simulink subsystem "ScanBlockwithDC"  (R2025b)
settings: Solver=VariableStepAuto  StartTime=0.0  StopTime=10.0  RelTol=1e-3
model mask{F0=grid.frequency, Theta0=0, Kp_LF=pll.kp, Ki_LF=pll.ki, Ts=5e-5, voltage=Base.KV_base_new, voltagedc=0, mva=0, Amplitude=0, Amplitude1=0, Amplitudedc=0, f=0, T=T, Tdis=5, Tend=10, VSelect=Equivalent Series Voltage (V), Hold=Yes}
  mask prompts: F0 "physmod:ee:library:comments:control:eeSinusoidalMeasurement:InitialFrequencyHz_MP"; Theta0 "physmod:ee:library:comments:control:eeSinusoidalMeasurement:InitialPhaseAnglerad_MP"; Kp_LF "physmod:ee:library:comments:control:eeSinusoidalMeasurement:LoopFilterProportionalGain_MP"; Ki_LF "physmod:ee:library:comments:control:eeSinusoidalMeasurement:LoopFilterIntegralGain_MP"; Ts "physmod:ee:library:comments:control:eeSinusoidalMeasurement:SampleTime1ForInherited_MP"; voltage "Base Voltage AC (Volts)"; voltagedc "Base Voltage DC (Volts)"; mva "Base Volt Ampere (VA)"; Amplitude "PRBS Magnitude Along Vd (PU)"; Amplitude1 "PRBS Magnitude Along Vq (PU)"; Amplitudedc "PRBS Magnitude Along Vdc (PU)"; f "Disturbance Frequency Vector (Hz)"; T "Sample Time of PRBS (sec)"; Tdis "Injection Start Time (sec)"; Tend "Injection End Time (sec)"; VSelect "Voltage Measuremnt Point"; Hold "Hold Frequency constant During Disturbance"
undefined symbols (not defined in the file or in its folder): DiscIntNeverNeededParam, ee_sli_rtmsupport, gcbh, w
libraries: slctrl_fre x12, ee_lib x5, eeGeneralControl x4, eeTransforms x4, nesl_utility x3, slctrl_signal x3, simulink x1
(part 1 of 3)
settings Model: Creator=rajarshd  LastModifiedBy=rajarshd
settings RTWCC: GPUComputeCapability=3.5

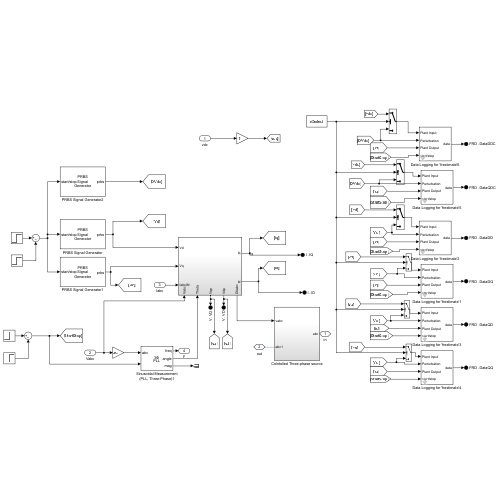
[thumbnail: Simulink's stored preview of the top-level diagram]
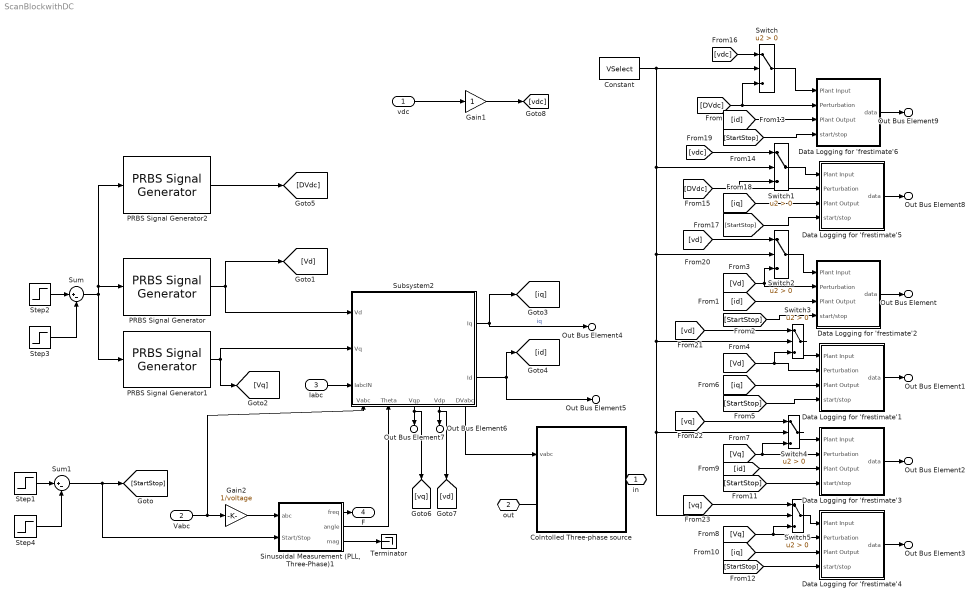
== system ScanBlockwithDC ==
  vdc : Inport
  Vabc : Inport  Port=2
  Iabc : Inport  Port=3
  Colntolled Three-phase source : Subsystem
  Constant : Constant  Value=VSelect
  Data Logging for 'frestimate'1 : Subsystem  mask(Companion Data Logger){Ts=T, SignalType=PRBS, Frequencies=[1:1:2e3], NumOfSetPeriod=1, NumOfEstPeriod=1, PRBSNumOfPeriod=1, ReadySignalActiveChoice=VariantPRBS, InfoSignalActiveChoice=VariantPRBS}
      mask prompts: Ts "Sample Time (Ts)"; SignalType "Input Signal Type"; Frequencies "Frequencies Vector"; NumOfSetPeriod "Number of Settling Periods"; NumOfEstPeriod "Number of Estimation Periods"; PRBSNumOfPeriod "Number of PRBS Signal Periods"; ReadySignalActiveChoice "Simulink:Variants:LabelComboBox"; InfoSignalActiveChoice "Simulink:Variants:LabelComboBox"
      mask help: Log data from signal generator blocks to work with "frestimate" API or frequency response estimation.
      mask init:
      | IsSinestreamSignal = strcmpi(get_param(gcb,'SignalType'),'Sinestream');
      |     IsPRBSSignal = strcmpi(get_param(gcb,'SignalType'),'PRBS');
      |     maskObj = Simulink.Mask.get(gcb);
      |     objectSinestream = maskObj.getDialogControl('SinestreamPanel');
      |     objectPRBS = maskObj.getDialogControl('PRBSPanel');
      |     %% Update optional inports
      |     inport_name = {'Frequency Index'};
      |     AvailableBlocks = get_param(gcb,'Blocks');
      |     % what exists in the block (old)
      |     type_in_block = ismember(inport_name,AvailableBlocks);
      |     % what is specified in the dialog (new)
      |     type_in_mask = IsSinestreamSignal;
      |     if IsSinestreamSignal
      |         objectSinestream.Visible = 'on';
      |         objectPRBS.Visible = 'off';
      |         set_param(gcb,'ReadySignalActiveChoice','VariantSinestream');  
      |         set_param(gcb,'InfoSignalActiveChoice','VariantSinestream');        
      |     elseif IsPRBSSignal
      |         objectSinestream.Visible = 'off';
      |         objectPRBS.Visible = 'on';
      |         set_param(gcb,'ReadySignalActiveChoice','VariantPRBS');  
      |         set_param(gcb,'InfoSignalActiveChoice','VariantPRBS');        
      |     end
      |     % Update Inport
      |     port = 5;
      |     %port = slctrlblkdlgs.OnlinePIDTuner.utilUpdateInport(gcb,'RateTransition_idx',AvailableBlocks,type_in_mask,type_in_block,1,'Frequency Index',port,1,'Frequencies','double');
      mask TypeOptions SignalType: Sinestream | PRBS
      mask TypeOptions ReadySignalActiveChoice: Generate Ready Signal/LabelModeActiveChoice
      mask TypeOptions InfoSignalActiveChoice: Generate Info Signal/LabelModeActiveChoice
      mask DialogControl Container3 Prompt: Signal Specific Settings
      mask DialogControl ReadySignalActiveChoice Prompt: Label mode active choice:
      mask DialogControl InfoSignalActiveChoice Prompt: Label mode active choice:
  Data Logging for 'frestimate'2 : Subsystem  mask(Companion Data Logger){Ts=T, SignalType=PRBS, Frequencies=[1:1:2e3], NumOfSetPeriod=1, NumOfEstPeriod=1, PRBSNumOfPeriod=1, ReadySignalActiveChoice=VariantPRBS, InfoSignalActiveChoice=VariantPRBS}
      mask prompts: Ts "Sample Time (Ts)"; SignalType "Input Signal Type"; Frequencies "Frequencies Vector"; NumOfSetPeriod "Number of Settling Periods"; NumOfEstPeriod "Number of Estimation Periods"; PRBSNumOfPeriod "Number of PRBS Signal Periods"; ReadySignalActiveChoice "Simulink:Variants:LabelComboBox"; InfoSignalActiveChoice "Simulink:Variants:LabelComboBox"
      mask help: Log data from signal generator blocks to work with "frestimate" API or frequency response estimation.
      mask init:
      | IsSinestreamSignal = strcmpi(get_param(gcb,'SignalType'),'Sinestream');
      |     IsPRBSSignal = strcmpi(get_param(gcb,'SignalType'),'PRBS');
      |     maskObj = Simulink.Mask.get(gcb);
      |     objectSinestream = maskObj.getDialogControl('SinestreamPanel');
      |     objectPRBS = maskObj.getDialogControl('PRBSPanel');
      |     %% Update optional inports
      |     inport_name = {'Frequency Index'};
      |     AvailableBlocks = get_param(gcb,'Blocks');
      |     % what exists in the block (old)
      |     type_in_block = ismember(inport_name,AvailableBlocks);
      |     % what is specified in the dialog (new)
      |     type_in_mask = IsSinestreamSignal;
      |     if IsSinestreamSignal
      |         objectSinestream.Visible = 'on';
      |         objectPRBS.Visible = 'off';
      |         set_param(gcb,'ReadySignalActiveChoice','VariantSinestream');  
      |         set_param(gcb,'InfoSignalActiveChoice','VariantSinestream');        
      |     elseif IsPRBSSignal
      |         objectSinestream.Visible = 'off';
      |         objectPRBS.Visible = 'on';
      |         set_param(gcb,'ReadySignalActiveChoice','VariantPRBS');  
      |         set_param(gcb,'InfoSignalActiveChoice','VariantPRBS');        
      |     end
      |     % Update Inport
      |     port = 5;
      |   %  port = slctrlblkdlgs.OnlinePIDTuner.utilUpdateInport(gcb,'RateTransition_idx',AvailableBlocks,type_in_mask,type_in_block,1,'Frequency Index',port,1,'Frequencies','double');
      mask TypeOptions SignalType: Sinestream | PRBS
      mask TypeOptions ReadySignalActiveChoice: Generate Ready Signal/LabelModeActiveChoice
      mask TypeOptions InfoSignalActiveChoice: Generate Info Signal/LabelModeActiveChoice
      mask DialogControl Container3 Prompt: Signal Specific Settings
      mask DialogControl ReadySignalActiveChoice Prompt: Label mode active choice:
      mask DialogControl InfoSignalActiveChoice Prompt: Label mode active choice:
  Data Logging for 'frestimate'3 : Subsystem  mask(Companion Data Logger){Ts=T, SignalType=PRBS, Frequencies=[1:1:2e3], NumOfSetPeriod=1, NumOfEstPeriod=1, PRBSNumOfPeriod=1, ReadySignalActiveChoice=VariantPRBS, InfoSignalActiveChoice=VariantPRBS}
      mask prompts: Ts "Sample Time (Ts)"; SignalType "Input Signal Type"; Frequencies "Frequencies Vector"; NumOfSetPeriod "Number of Settling Periods"; NumOfEstPeriod "Number of Estimation Periods"; PRBSNumOfPeriod "Number of PRBS Signal Periods"; ReadySignalActiveChoice "Simulink:Variants:LabelComboBox"; InfoSignalActiveChoice "Simulink:Variants:LabelComboBox"
      mask help: Log data from signal generator blocks to work with "frestimate" API or frequency response estimation.
      mask init: same as ScanBlockwithDC/Data Logging for 'frestimate'1
      mask TypeOptions SignalType: Sinestream | PRBS
      mask TypeOptions ReadySignalActiveChoice: Generate Ready Signal/LabelModeActiveChoice
      mask TypeOptions InfoSignalActiveChoice: Generate Info Signal/LabelModeActiveChoice
      mask DialogControl Container3 Prompt: Signal Specific Settings
      mask DialogControl ReadySignalActiveChoice Prompt: Label mode active choice:
      mask DialogControl InfoSignalActiveChoice Prompt: Label mode active choice:
  Data Logging for 'frestimate'4 : Subsystem  mask(Companion Data Logger){Ts=T, SignalType=PRBS, Frequencies=[1:1:2e3], NumOfSetPeriod=1, NumOfEstPeriod=1, PRBSNumOfPeriod=1, ReadySignalActiveChoice=VariantPRBS, InfoSignalActiveChoice=VariantPRBS}
      mask prompts: Ts "Sample Time (Ts)"; SignalType "Input Signal Type"; Frequencies "Frequencies Vector"; NumOfSetPeriod "Number of Settling Periods"; NumOfEstPeriod "Number of Estimation Periods"; PRBSNumOfPeriod "Number of PRBS Signal Periods"; ReadySignalActiveChoice "Simulink:Variants:LabelComboBox"; InfoSignalActiveChoice "Simulink:Variants:LabelComboBox"
      mask help: Log data from signal generator blocks to work with "frestimate" API or frequency response estimation.
      mask init: same as ScanBlockwithDC/Data Logging for 'frestimate'1
      mask TypeOptions SignalType: Sinestream | PRBS
      mask TypeOptions ReadySignalActiveChoice: Generate Ready Signal/LabelModeActiveChoice
      mask TypeOptions InfoSignalActiveChoice: Generate Info Signal/LabelModeActiveChoice
      mask DialogControl Container3 Prompt: Signal Specific Settings
      mask DialogControl ReadySignalActiveChoice Prompt: Label mode active choice:
      mask DialogControl InfoSignalActiveChoice Prompt: Label mode active choice:
  Data Logging for 'frestimate'5 : Subsystem  mask(Companion Data Logger){Ts=T, SignalType=PRBS, Frequencies=[1:1:2e3], NumOfSetPeriod=1, NumOfEstPeriod=1, PRBSNumOfPeriod=1, ReadySignalActiveChoice=VariantPRBS, InfoSignalActiveChoice=VariantPRBS}
      mask prompts: Ts "Sample Time (Ts)"; SignalType "Input Signal Type"; Frequencies "Frequencies Vector"; NumOfSetPeriod "Number of Settling Periods"; NumOfEstPeriod "Number of Estimation Periods"; PRBSNumOfPeriod "Number of PRBS Signal Periods"; ReadySignalActiveChoice "Simulink:Variants:LabelComboBox"; InfoSignalActiveChoice "Simulink:Variants:LabelComboBox"
      mask help: Log data from signal generator blocks to work with "frestimate" API or frequency response estimation.
      mask init:
      | IsSinestreamSignal = strcmpi(get_param(gcb,'SignalType'),'Sinestream');
      |     IsPRBSSignal = strcmpi(get_param(gcb,'SignalType'),'PRBS');
      |     maskObj = Simulink.Mask.get(gcb);
      |     objectSinestream = maskObj.getDialogControl('SinestreamPanel');
      |     objectPRBS = maskObj.getDialogControl('PRBSPanel');
      |     %% Update optional inports
      |     inport_name = {'Frequency Index'};
      |     AvailableBlocks = get_param(gcb,'Blocks');
      |     % what exists in the block (old)
      |     type_in_block = ismember(inport_name,AvailableBlocks);
      |     % what is specified in the dialog (new)
      |     type_in_mask = IsSinestreamSignal;
      |     if IsSinestreamSignal
      |         objectSinestream.Visible = 'on';
      |         objectPRBS.Visible = 'off';
      |         set_param(gcb,'ReadySignalActiveChoice','VariantSinestream');  
      |         set_param(gcb,'InfoSignalActiveChoice','VariantSinestream');        
      |     elseif IsPRBSSignal
      |         objectSinestream.Visible = 'off';
      |         objectPRBS.Visible = 'on';
      |         set_param(gcb,'ReadySignalActiveChoice','VariantPRBS');  
      |         set_param(gcb,'InfoSignalActiveChoice','VariantPRBS');        
      |     end
      |     % Update Inport
      |     port = 5;
      |    % port = slctrlblkdlgs.OnlinePIDTuner.utilUpdateInport(gcb,'RateTransition_idx',AvailableBlocks,type_in_mask,type_in_block,1,'Frequency Index',port,1,'Frequencies','double');
      mask TypeOptions SignalType: Sinestream | PRBS
      mask TypeOptions ReadySignalActiveChoice: Generate Ready Signal/LabelModeActiveChoice
      mask TypeOptions InfoSignalActiveChoice: Generate Info Signal/LabelModeActiveChoice
      mask DialogControl Container3 Prompt: Signal Specific Settings
      mask DialogControl ReadySignalActiveChoice Prompt: Label mode active choice:
      mask DialogControl InfoSignalActiveChoice Prompt: Label mode active choice:
  Data Logging for 'frestimate'6 : Subsystem  mask(Companion Data Logger){Ts=T, SignalType=PRBS, Frequencies=[1:1:2e3], NumOfSetPeriod=1, NumOfEstPeriod=1, PRBSNumOfPeriod=1, ReadySignalActiveChoice=VariantPRBS, InfoSignalActiveChoice=VariantPRBS}
      mask prompts: Ts "Sample Time (Ts)"; SignalType "Input Signal Type"; Frequencies "Frequencies Vector"; NumOfSetPeriod "Number of Settling Periods"; NumOfEstPeriod "Number of Estimation Periods"; PRBSNumOfPeriod "Number of PRBS Signal Periods"; ReadySignalActiveChoice "Simulink:Variants:LabelComboBox"; InfoSignalActiveChoice "Simulink:Variants:LabelComboBox"
      mask help: Log data from signal generator blocks to work with "frestimate" API or frequency response estimation.
      mask init: same as ScanBlockwithDC/Data Logging for 'frestimate'5
      mask TypeOptions SignalType: Sinestream | PRBS
      mask TypeOptions ReadySignalActiveChoice: Generate Ready Signal/LabelModeActiveChoice
      mask TypeOptions InfoSignalActiveChoice: Generate Info Signal/LabelModeActiveChoice
      mask DialogControl Container3 Prompt: Signal Specific Settings
      mask DialogControl ReadySignalActiveChoice Prompt: Label mode active choice:
      mask DialogControl InfoSignalActiveChoice Prompt: Label mode active choice:
  Gain1 : Gain
  Gain2 : Gain  Gain=1/voltage
  PRBS Signal Generator : slctrl_signal/PRBS Signal Generator  DiscreteTs=T  BlockDataType=double  SignalSource=Block parameters  Frequencies=f*2*pi  FreqUnits=rad/s  Amplitudes=Amplitude*voltage+1e-9  NumOfFreq=3  NumOfPRBSPeriod=1  UseAutogenNumOfPRBSPeriod=off  PRBSSignalOrder=16  UseAutogenPRBSSignalOrder=on  UseExternalTs=off  CompiledTsChoice=InternalTs
      settings: LibrarySourceBlock=slctrlblks/Signal Generation/PRBS Signal Generator
  PRBS Signal Generator1 : slctrl_signal/PRBS Signal Generator  DiscreteTs=T  BlockDataType=double  SignalSource=Block parameters  Frequencies=f*2*pi  FreqUnits=rad/s  Amplitudes=Amplitude1*voltage+1e-9  NumOfFreq=3  NumOfPRBSPeriod=1  UseAutogenNumOfPRBSPeriod=off  PRBSSignalOrder=16  UseAutogenPRBSSignalOrder=on  UseExternalTs=off  CompiledTsChoice=InternalTs
      settings: LibrarySourceBlock=slctrlblks/Signal Generation/PRBS Signal Generator
  PRBS Signal Generator2 : slctrl_signal/PRBS Signal Generator  DiscreteTs=T  BlockDataType=double  SignalSource=Block parameters  Frequencies=f*2*pi  FreqUnits=rad/s  Amplitudes=Amplitudedc*voltagedc+1e-9  NumOfFreq=3  NumOfPRBSPeriod=1  UseAutogenNumOfPRBSPeriod=off  PRBSSignalOrder=16  UseAutogenPRBSSignalOrder=on  UseExternalTs=off  CompiledTsChoice=InternalTs
      settings: LibrarySourceBlock=slctrlblks/Signal Generation/PRBS Signal Generator
  "Sinusoidal Measurement (PLL, Three-Phase)1" : Subsystem  LoadFcn=ee_sli_rtmsupport( 'loadfcn', gcbh );  mask(Sinusoidal Measurement (PLL, Three-Phase)){Kp_LF=Kp_LF, Ki_LF=Ki_LF, F0=F0, Theta0=Theta0, Ts=Ts}
      mask prompts: Kp_LF "physmod:ee:library:comments:control:eeSinusoidalMeasurement:LoopFilterProportionalGain_MP"; Ki_LF "physmod:ee:library:comments:control:eeSinusoidalMeasurement:LoopFilterIntegralGain_MP"; F0 "physmod:ee:library:comments:control:eeSinusoidalMeasurement:InitialFrequencyHz_MP"; Theta0 "physmod:ee:library:comments:control:eeSinusoidalMeasurement:InitialPhaseAnglerad_MP"; Ts "physmod:ee:library:comments:control:eeSinusoidalMeasurement:SampleTime1ForInherited_MP"
      mask help: physmod:ee:library:comments:control:eeSinusoidalMeasurement:SinusoidalPowerMeasurementPLLThreePhase_MD
      mask init:
      | timeDomain = ee.mask.initializeThreePhaseSinusoidalMeasurementPLL(Ts);
      settings: CopyFcn=ee_sli_rtmsupport( 'copyfcn', gcbh );  DeleteFcn=ee_sli_rtmsupport( 'deletefcn', gcbh );  ModelCloseFcn=ee_sli_rtmsupport( 'modelclosefcn', gcbh );  PostSaveFcn=ee_sli_rtmsupport( 'postsavefcn', gcbh );  PreCopyFcn=ee_sli_rtmsupport( 'precopyfcn', gcbh );  OpenFcn=ee_sli_rtmsupport( 'openfcn', gcbh );  CloseFcn=ee_sli_rtmsupport( 'closefcn', gcbh );  PreDeleteFcn=ee_sli_rtmsupport( 'predeletefcn', gcbh );
      settings: LibrarySourceBlock=|
      | ee_sl_lib/Measurements/Sinusoidal Measurement
      | (PLL, Three-Phase)
      mask Help: web(nesl_help(gcbh))
      mask TypeOptions Ts:
      | Angle/Integrator with
      | Wrapped State
      | (Discrete or Continuous)/Ts | PI/Integrator
      | (Discrete or Continuous)/Ts | Moving Average
      | (Variable Frequency)/Ts | Low-Pass Filter
      | (Discrete or Continuous)/Ts
      mask DialogControl Kp_LF Prompt: Loop filter proportional gain
      mask DialogControl Ki_LF Prompt: Loop filter integral gain
      mask DialogControl F0 Prompt: Initial frequency (Hz)
      mask DialogControl Theta0 Prompt: Initial phase angle (rad)
      mask DialogControl Ts Prompt: Sample time (-1 for inherited)
      mask Display: ee.mask.drawThreePhaseSinusoidalMeasurementPLL;
  Step1 : Step  Time=Tdis-0.001  SampleTime=Ts
  Step2 : Step  Time=Tdis  SampleTime=Ts
  Step3 : Step  Time=Tend  SampleTime=Ts
  Step4 : Step  Time=Tend-0.001  SampleTime=Ts
  Subsystem2 : Subsystem
      settings: PortSchema="{\"entries\":[{\"content\":{\"sides\":[{\"content\":{\"connectorIds\":[\"In1\",\"In2\",\"In3\"]},\"type\":\"ConnectorPlacement.EquallySpacedRectSide\",\"uuid\":\"9594ab20-6a90-4061-9191-964719779161\"},{\"content\":{\"connectorIds\":[\"Out1\",\"Out2\"],\"side\":\"RIGHT\"},\"type\":\"ConnectorPlacement.EquallySpacedRectSide\",\"uuid\":\"7728c146-30c2-48f5-81ca-653b56ee64fb\"},{\"content\":{\"side\":\"TOP\"},\"type\":\"ConnectorPlacement.EquallySpacedRectSide\",\"uuid\":\"8060c2dd-01d9-4157-a0b3-59db77887fcf\"},{\"content\":{\"connectorIds\":[\"In4\",\"In5\",\"Out3\",\"Out4\",\"Out5\"],\"side\":\"BOTTOM\"},\"type\":\"ConnectorPlacement.EquallySpacedRectSide\",\"uuid\":\"6c62adf9-210a-4ad7-b383-6cff41840c61\"}]},\"type\":\"ConnectorPlacement.EquallySpacedConnector\",\"uuid\":\"38a4dacf-dba1-4794-be83-b6cd11059d5d\"}],\"packageUris\":[\"http://schema.mathworks.com/mf0/Connector/R2020b\"],\"version\":\"1.0\"}"
  Sum : Sum  Inputs=|+-
  Sum1 : Sum  Inputs=|+-
  Switch{,1..5} (6 alike) : Switch  Criteria=u2 > Threshold  SaturateOnIntegerOverflow=off  InputSameDT=off
  Terminator : Terminator
  in : PMIOPort  Side=Left
  out : PMIOPort  Port=2  Side=Right
  Out Bus Element : Outport  PortName=FRD  Element=DataDD
  Out Bus Element1 : Outport  PortName=FRD  Element=DataDQ
  Out Bus Element2 : Outport  PortName=FRD  Element=DataQD
  Out Bus Element3 : Outport  PortName=FRD  Element=DataQQ
  Out Bus Element8 : Outport  PortName=FRD  Element=DataQDC
  Out Bus Element9 : Outport  PortName=FRD  Element=DataDDC
  Out Bus Element4 : Outport  Port=2  PortName=I  Element=IQ
  Out Bus Element5 : Outport  Port=2  PortName=I  Element=ID
  Out Bus Element6 : Outport  Port=3  PortName=V  Element=VD
  Out Bus Element7 : Outport  Port=3  PortName=V  Element=VQ
  F : Outport  Port=4  SampleTime=Ts
  wires:
  PRBS Signal Generator1/1 -> Subsystem2/2(Vq), [Vq]
  "Sinusoidal Measurement (PLL, Three-Phase)1"/1(freq) -> F/1
  Subsystem2/5(DVabc) -> Colntolled Three-phase source/1(vabc)
  "Sinusoidal Measurement (PLL, Three-Phase)1"/2(angle) -> Subsystem2/5(Theta)
  Subsystem2/1(Iq) -> [iq], Out Bus Element4/1  "iq"
  Subsystem2/2(Id) -> [id], Out Bus Element5/1
  "Sinusoidal Measurement (PLL, Three-Phase)1"/3(mag) -> Terminator/1
  Step2/1 -> Sum/1
  Sum/1 -> PRBS Signal Generator1/1, PRBS Signal Generator/1, PRBS Signal Generator2/1
  Step3/1 -> Sum/2
  PRBS Signal Generator/1 -> Subsystem2/1(Vd), [Vd]
  [id] -> Data Logging for 'frestimate'2/3(Plant Output)
  [StartStop] -> Data Logging for 'frestimate'2/4(start/stop)
  [StartStop] -> Data Logging for 'frestimate'1/4(start/stop)
  [iq] -> Data Logging for 'frestimate'1/3(Plant Output)
  [id] -> Data Logging for 'frestimate'3/3(Plant Output)
  [iq] -> Data Logging for 'frestimate'4/3(Plant Output)
  [StartStop] -> Data Logging for 'frestimate'3/4(start/stop)
  [StartStop] -> Data Logging for 'frestimate'4/4(start/stop)
  Step4/1 -> Sum1/2
  Step1/1 -> Sum1/1
  Subsystem2/4(Vdp) -> Out Bus Element6/1, [vd]
  Subsystem2/3(Vqp) -> Out Bus Element7/1, [vq]
  Iabc/1 -> Subsystem2/3(IabcIN)
  Data Logging for 'frestimate'2/1(data) -> Out Bus Element/1
  Data Logging for 'frestimate'1/1(data) -> Out Bus Element1/1
  Data Logging for 'frestimate'3/1(data) -> Out Bus Element2/1
  Data Logging for 'frestimate'4/1(data) -> Out Bus Element3/1
  Sum1/1 -> [StartStop], "Sinusoidal Measurement (PLL, Three-Phase)1"/2(Start/Stop)
  Data Logging for 'frestimate'5/1(data) -> Out Bus Element8/1
  Data Logging for 'frestimate'6/1(data) -> Out Bus Element9/1
  [iq] -> Data Logging for 'frestimate'5/3(Plant Output)
  [StartStop] -> Data Logging for 'frestimate'5/4(start/stop)
  [id] -> Data Logging for 'frestimate'6/3(Plant Output)
  [StartStop] -> Data Logging for 'frestimate'6/4(start/stop)
  PRBS Signal Generator2/1 -> [DVdc]
  [DVdc] -> Data Logging for 'frestimate'6/2(Perturbation), Switch/3
  [DVdc] -> Data Logging for 'frestimate'5/2(Perturbation), Switch1/3
  vdc/1 -> Gain1/1
  [Vd] -> Switch2/3, Data Logging for 'frestimate'2/2(Perturbation)
  [Vd] -> Data Logging for 'frestimate'1/2(Perturbation), Switch3/3
  [Vq] -> Data Logging for 'frestimate'3/2(Perturbation), Switch4/3
  [Vq] -> Data Logging for 'frestimate'4/2(Perturbation), Switch5/3
  Vabc/1 -> Subsystem2/4(Vabc), Gain2/1
  Gain1/1 -> [vdc]
  Gain2/1 -> "Sinusoidal Measurement (PLL, Three-Phase)1"/1(abc)
  [vdc] -> Switch/1
  Switch/1 -> Data Logging for 'frestimate'6/1(Plant Input)
  Switch1/1 -> Data Logging for 'frestimate'5/1(Plant Input)
  [vdc] -> Switch1/1
  Constant/1 -> Switch/2, Switch1/2, Switch3/2, Switch5/2, Switch4/2, Switch2/2
  [vd] -> Switch2/1
  Switch2/1 -> Data Logging for 'frestimate'2/1(Plant Input)
  Switch3/1 -> Data Logging for 'frestimate'1/1(Plant Input)
  [vd] -> Switch3/1
  Switch4/1 -> Data Logging for 'frestimate'3/1(Plant Input)
  [vq] -> Switch4/1
  Switch5/1 -> Data Logging for 'frestimate'4/1(Plant Input)
  [vq] -> Switch5/1
  connections:
  Colntolled Three-phase source/RConn1 -- in/RConn1
  out/RConn1 -- Colntolled Three-phase source/LConn1

== system ScanBlockwithDC/Colntolled Three-phase source ==
  vabc : Inport
  Demux : Demux  Outputs=3
  Phase Splitter : ee_lib/Connectors & References/Phase Splitter
  Phase Splitter1 : ee_lib/Connectors & References/Phase Splitter
  Programmable Voltage Source : ee_lib/Sources/Programmable Voltage Source  magnitude_type=ee.enum.timechanging.constant  ac_magnitude=0 V  magn_ramp=1 V/s  magn_step=1 V  magn_modu_magn=1 V  magn_modu_freq=1 Hz  magn_t1=1 s  magn_t2=2 s  frequency_type=ee.enum.timechanging.constant  ac_frequency=60 Hz  freq_ramp=1 Hz/s  freq_step=1 Hz  freq_modu_magn=1 Hz  freq_modu_freq=1 Hz  freq_t1=1 s  freq_t2=2 s  phase_type=ee.enum.timechanging.constant  ac_shift=0 deg  phase_ramp=1 deg/s  phase_step=1 deg  phase_modu_magn=1 deg  phase_modu_freq=1 Hz  phase_t1=1 s  phase_t2=2 s  dc_type=ee.enum.timechanging.external  dc_voltage=0 V  dc_ramp=1 V/s  dc_step=1 V  dc_modu_magn=1 V  dc_modu_freq=1 Hz  dc_t1=1 s  dc_t2=2 s  harmonic_option=0  harmonic_orders=[5, 7, 11, 13]  harmonic_ratios=[.1, .1, .1, .1]  harmonic_shifts=[0, 0, 0, 0] deg  harmonic_t1=-inf s  harmonic_t2=inf s  noise_mode=0  PSD=0 V^2/Hz  repeatability=1  auto_seed=0  user_seed=0  sample_time=1e-3 s  i_specify=off  i_priority=None  i=0 A  i_nominal_specify=off  i_nominal_value=1  i_nominal_unit=A  v_specify=off  v_priority=None  v=0 V  v_nominal_specify=off  v_nominal_value=1  v_nominal_unit=V
      settings: InternalSimscapePortConfiguration="{\"Bottom\":[],\"Left\":[{\"id\":\"p\",\"label\":\"+\",\"type\":\"foundation.electrical.electrical\"}],\"Right\":[{\"id\":\"ext_dc\",\"label\":\"DC\",\"type\":\"input\"},{\"id\":\"n\",\"label\":\"-\",\"type\":\"foundation.electrical.electrical\"}],\"Top\":[]}"
  Programmable Voltage Source1 : ee_lib/Sources/Programmable Voltage Source  magnitude_type=ee.enum.timechanging.constant  ac_magnitude=0 V  magn_ramp=1 V/s  magn_step=1 V  magn_modu_magn=1 V  magn_modu_freq=1 Hz  magn_t1=1 s  magn_t2=2 s  frequency_type=ee.enum.timechanging.constant  ac_frequency=60 Hz  freq_ramp=1 Hz/s  freq_step=1 Hz  freq_modu_magn=1 Hz  freq_modu_freq=1 Hz  freq_t1=1 s  freq_t2=2 s  phase_type=ee.enum.timechanging.constant  ac_shift=0 deg  phase_ramp=1 deg/s  phase_step=1 deg  phase_modu_magn=1 deg  phase_modu_freq=1 Hz  phase_t1=1 s  phase_t2=2 s  dc_type=ee.enum.timechanging.external  dc_voltage=0 V  dc_ramp=1 V/s  dc_step=1 V  dc_modu_magn=1 V  dc_modu_freq=1 Hz  dc_t1=1 s  dc_t2=2 s  harmonic_option=0  harmonic_orders=[5, 7, 11, 13]  harmonic_ratios=[.1, .1, .1, .1]  harmonic_shifts=[0, 0, 0, 0] deg  harmonic_t1=-inf s  harmonic_t2=inf s  noise_mode=0  PSD=0 V^2/Hz  repeatability=1  auto_seed=0  user_seed=0  sample_time=1e-3 s  i_specify=off  i_priority=None  i=0 A  i_nominal_specify=off  i_nominal_value=1  i_nominal_unit=A  v_specify=off  v_priority=None  v=0 V  v_nominal_specify=off  v_nominal_value=1  v_nominal_unit=V
      settings: InternalSimscapePortConfiguration="{\"Bottom\":[],\"Left\":[{\"id\":\"p\",\"label\":\"+\",\"type\":\"foundation.electrical.electrical\"}],\"Right\":[{\"id\":\"ext_dc\",\"label\":\"DC\",\"type\":\"input\"},{\"id\":\"n\",\"label\":\"-\",\"type\":\"foundation.electrical.electrical\"}],\"Top\":[]}"
  Programmable Voltage Source2 : ee_lib/Sources/Programmable Voltage Source  magnitude_type=ee.enum.timechanging.constant  ac_magnitude=0 V  magn_ramp=1 V/s  magn_step=1 V  magn_modu_magn=1 V  magn_modu_freq=1 Hz  magn_t1=1 s  magn_t2=2 s  frequency_type=ee.enum.timechanging.constant  ac_frequency=60 Hz  freq_ramp=1 Hz/s  freq_step=1 Hz  freq_modu_magn=1 Hz  freq_modu_freq=1 Hz  freq_t1=1 s  freq_t2=2 s  phase_type=ee.enum.timechanging.constant  ac_shift=0 deg  phase_ramp=1 deg/s  phase_step=1 deg  phase_modu_magn=1 deg  phase_modu_freq=1 Hz  phase_t1=1 s  phase_t2=2 s  dc_type=ee.enum.timechanging.external  dc_voltage=0 V  dc_ramp=1 V/s  dc_step=1 V  dc_modu_magn=1 V  dc_modu_freq=1 Hz  dc_t1=1 s  dc_t2=2 s  harmonic_option=0  harmonic_orders=[5, 7, 11, 13]  harmonic_ratios=[.1, .1, .1, .1]  harmonic_shifts=[0, 0, 0, 0] deg  harmonic_t1=-inf s  harmonic_t2=inf s  noise_mode=0  PSD=0 V^2/Hz  repeatability=1  auto_seed=0  user_seed=0  sample_time=1e-3 s  i_specify=off  i_priority=None  i=0 A  i_nominal_specify=off  i_nominal_value=1  i_nominal_unit=A  v_specify=off  v_priority=None  v=0 V  v_nominal_specify=off  v_nominal_value=1  v_nominal_unit=V
      settings: InternalSimscapePortConfiguration="{\"Bottom\":[],\"Left\":[{\"id\":\"p\",\"label\":\"+\",\"type\":\"foundation.electrical.electrical\"}],\"Right\":[{\"id\":\"ext_dc\",\"label\":\"DC\",\"type\":\"input\"},{\"id\":\"n\",\"label\":\"-\",\"type\":\"foundation.electrical.electrical\"}],\"Top\":[]}"
  Simulink-PS Converter : nesl_utility/Simulink-PS Converter  PhysicalDomain=network_engine_domain  SubClassName=ps_input  LeftPortType=input  RightPortType=output  PseudoPeriodic=off  Frequencies=[]  NoiseDistribution=none  NoiseParameters=[]  Unit=1  AffineConversion=off  FilteringAndDerivatives=provide  SimscapeFilterOrder=1  InputFilterTimeConstant=0.001  UdotUserProvided=0
  Simulink-PS Converter1 : nesl_utility/Simulink-PS Converter  PhysicalDomain=network_engine_domain  SubClassName=ps_input  LeftPortType=input  RightPortType=output  PseudoPeriodic=off  Frequencies=[]  NoiseDistribution=none  NoiseParameters=[]  Unit=1  AffineConversion=off  FilteringAndDerivatives=provide  SimscapeFilterOrder=1  InputFilterTimeConstant=0.001  UdotUserProvided=0
  Simulink-PS Converter2 : nesl_utility/Simulink-PS Converter  PhysicalDomain=network_engine_domain  SubClassName=ps_input  LeftPortType=input  RightPortType=output  PseudoPeriodic=off  Frequencies=[]  NoiseDistribution=none  NoiseParameters=[]  Unit=1  AffineConversion=off  FilteringAndDerivatives=provide  SimscapeFilterOrder=1  InputFilterTimeConstant=0.001  UdotUserProvided=0
  abc1 : PMIOPort  Side=Left
  abc : PMIOPort  Port=2  Side=Right
  wires:
  Demux/1 -> Simulink-PS Converter2/1
  Demux/2 -> Simulink-PS Converter1/1
  Demux/3 -> Simulink-PS Converter/1
  vabc/1 -> Demux/1
  connections:
  abc1/RConn1 -- Phase Splitter/LConn1
  Simulink-PS Converter2/RConn1 -- Programmable Voltage Source/RConn1
  Simulink-PS Converter1/RConn1 -- Programmable Voltage Source1/RConn1
  Simulink-PS Converter/RConn1 -- Programmable Voltage Source2/RConn1
  Phase Splitter1/LConn1 -- abc/RConn1
  Programmable Voltage Source1/RConn2 -- Phase Splitter1/RConn2
  Programmable Voltage Source1/LConn1 -- Phase Splitter/RConn2
  Programmable Voltage Source/LConn1 -- Phase Splitter/RConn1
  Programmable Voltage Source/RConn2 -- Phase Splitter1/RConn1
  Programmable Voltage Source2/RConn2 -- Phase Splitter1/RConn3
  Programmable Voltage Source2/LConn1 -- Phase Splitter/RConn3

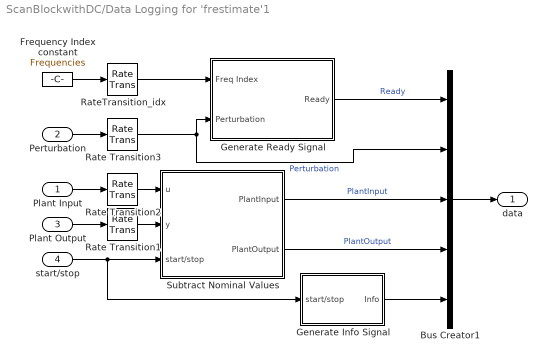
== system ScanBlockwithDC/Data Logging for 'frestimate'1 ==
  Plant Input : Inport
  Perturbation : Inport  Port=2
  Plant Output : Inport  Port=3
  start/stop : Inport  Port=4
  Bus Creator1 : BusCreator  Inputs=5
  Frequency Index constant : Constant  Value=Frequencies  OutDataTypeStr=double
  Generate Info Signal : Subsystem  Variant=on  VariantControlMode=label  LabelModeActiveChoice=VariantPRBS
  Generate Ready Signal : Subsystem  Variant=on  VariantControlMode=label  LabelModeActiveChoice=VariantPRBS
  Rate Transition1 : RateTransition  OutPortSampleTime=Ts
  Rate Transition2 : RateTransition  OutPortSampleTime=Ts
  Rate Transition3 : RateTransition  OutPortSampleTime=Ts
  RateTransition_idx : RateTransition  OutPortSampleTime=Ts
  Subtract Nominal Values : Subsystem
  data : Outport
  wires:
  Frequency Index constant/1 -> RateTransition_idx/1
  RateTransition_idx/1 -> Generate Ready Signal/1(Freq Index)
  Perturbation/1 -> Rate Transition3/1
  Rate Transition1/1 -> Subtract Nominal Values/2(y)
  Rate Transition2/1 -> Subtract Nominal Values/1(u)
  start/stop/1 -> Subtract Nominal Values/3(start/stop), Generate Info Signal/1(start/stop)
  Plant Input/1 -> Rate Transition2/1
  Plant Output/1 -> Rate Transition1/1
  Generate Ready Signal/1(Ready) -> Bus Creator1/1  "Ready"
  Subtract Nominal Values/2(PlantOutput) -> Bus Creator1/4  "PlantOutput"
  Subtract Nominal Values/1(PlantInput) -> Bus Creator1/3  "PlantInput"
  Rate Transition3/1 -> Bus Creator1/2, Generate Ready Signal/2(Perturbation)  "Perturbation"
  Bus Creator1/1 -> data/1
  Generate Info Signal/1(Info) -> Bus Creator1/5

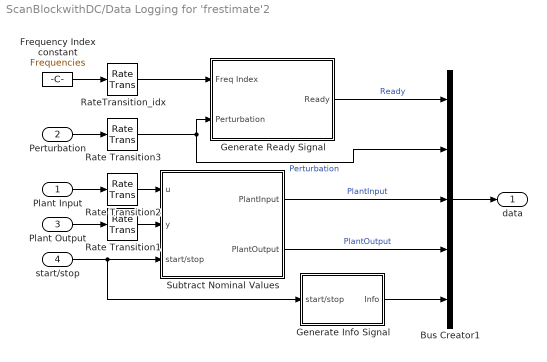
== system ScanBlockwithDC/Data Logging for 'frestimate'2 ==
  Plant Input : Inport
  Perturbation : Inport  Port=2
  Plant Output : Inport  Port=3
  start/stop : Inport  Port=4
  Bus Creator1 : BusCreator  Inputs=5
  Frequency Index constant : Constant  Value=Frequencies  OutDataTypeStr=double
  Generate Info Signal : Subsystem  Variant=on  VariantControlMode=label  LabelModeActiveChoice=VariantPRBS
  Generate Ready Signal : Subsystem  Variant=on  VariantControlMode=label  LabelModeActiveChoice=VariantPRBS
  Rate Transition1 : RateTransition  OutPortSampleTime=Ts
  Rate Transition2 : RateTransition  OutPortSampleTime=Ts
  Rate Transition3 : RateTransition  OutPortSampleTime=Ts
  RateTransition_idx : RateTransition  OutPortSampleTime=Ts
  Subtract Nominal Values : Subsystem
  data : Outport
  wires:
  Frequency Index constant/1 -> RateTransition_idx/1
  RateTransition_idx/1 -> Generate Ready Signal/1(Freq Index)
  Perturbation/1 -> Rate Transition3/1
  Rate Transition1/1 -> Subtract Nominal Values/2(y)
  Rate Transition2/1 -> Subtract Nominal Values/1(u)
  start/stop/1 -> Subtract Nominal Values/3(start/stop), Generate Info Signal/1(start/stop)
  Plant Input/1 -> Rate Transition2/1
  Plant Output/1 -> Rate Transition1/1
  Generate Ready Signal/1(Ready) -> Bus Creator1/1  "Ready"
  Subtract Nominal Values/2(PlantOutput) -> Bus Creator1/4  "PlantOutput"
  Subtract Nominal Values/1(PlantInput) -> Bus Creator1/3  "PlantInput"
  Rate Transition3/1 -> Bus Creator1/2, Generate Ready Signal/2(Perturbation)  "Perturbation"
  Bus Creator1/1 -> data/1
  Generate Info Signal/1(Info) -> Bus Creator1/5

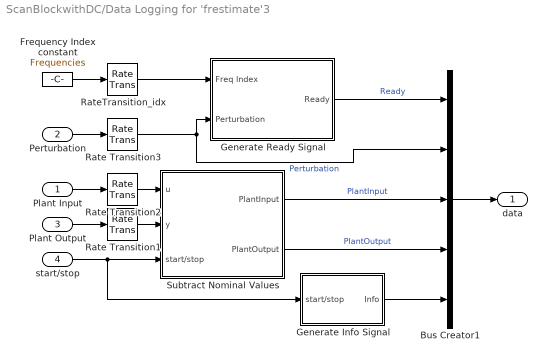
== system ScanBlockwithDC/Data Logging for 'frestimate'3 ==
  Plant Input : Inport
  Perturbation : Inport  Port=2
  Plant Output : Inport  Port=3
  start/stop : Inport  Port=4
  Bus Creator1 : BusCreator  Inputs=5
  Frequency Index constant : Constant  Value=Frequencies  OutDataTypeStr=double
  Generate Info Signal : Subsystem  Variant=on  VariantControlMode=label  LabelModeActiveChoice=VariantPRBS
  Generate Ready Signal : Subsystem  Variant=on  VariantControlMode=label  LabelModeActiveChoice=VariantPRBS
  Rate Transition1 : RateTransition  OutPortSampleTime=Ts
  Rate Transition2 : RateTransition  OutPortSampleTime=Ts
  Rate Transition3 : RateTransition  OutPortSampleTime=Ts
  RateTransition_idx : RateTransition  OutPortSampleTime=Ts
  Subtract Nominal Values : Subsystem
  data : Outport
  wires:
  Frequency Index constant/1 -> RateTransition_idx/1
  RateTransition_idx/1 -> Generate Ready Signal/1(Freq Index)
  Perturbation/1 -> Rate Transition3/1
  Rate Transition1/1 -> Subtract Nominal Values/2(y)
  Rate Transition2/1 -> Subtract Nominal Values/1(u)
  start/stop/1 -> Subtract Nominal Values/3(start/stop), Generate Info Signal/1(start/stop)
  Plant Input/1 -> Rate Transition2/1
  Plant Output/1 -> Rate Transition1/1
  Generate Ready Signal/1(Ready) -> Bus Creator1/1  "Ready"
  Subtract Nominal Values/2(PlantOutput) -> Bus Creator1/4  "PlantOutput"
  Subtract Nominal Values/1(PlantInput) -> Bus Creator1/3  "PlantInput"
  Rate Transition3/1 -> Bus Creator1/2, Generate Ready Signal/2(Perturbation)  "Perturbation"
  Bus Creator1/1 -> data/1
  Generate Info Signal/1(Info) -> Bus Creator1/5

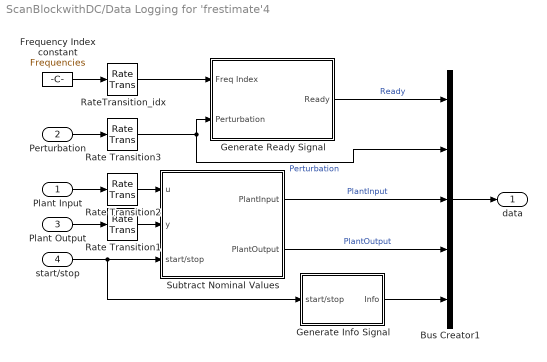
== system ScanBlockwithDC/Data Logging for 'frestimate'4 ==
  Plant Input : Inport
  Perturbation : Inport  Port=2
  Plant Output : Inport  Port=3
  start/stop : Inport  Port=4
  Bus Creator1 : BusCreator  Inputs=5
  Frequency Index constant : Constant  Value=Frequencies  OutDataTypeStr=double
  Generate Info Signal : Subsystem  Variant=on  VariantControlMode=label  LabelModeActiveChoice=VariantPRBS
  Generate Ready Signal : Subsystem  Variant=on  VariantControlMode=label  LabelModeActiveChoice=VariantPRBS
  Rate Transition1 : RateTransition  OutPortSampleTime=Ts
  Rate Transition2 : RateTransition  OutPortSampleTime=Ts
  Rate Transition3 : RateTransition  OutPortSampleTime=Ts
  RateTransition_idx : RateTransition  OutPortSampleTime=Ts
  Subtract Nominal Values : Subsystem
  data : Outport
  wires:
  Frequency Index constant/1 -> RateTransition_idx/1
  RateTransition_idx/1 -> Generate Ready Signal/1(Freq Index)
  Perturbation/1 -> Rate Transition3/1
  Rate Transition1/1 -> Subtract Nominal Values/2(y)
  Rate Transition2/1 -> Subtract Nominal Values/1(u)
  start/stop/1 -> Subtract Nominal Values/3(start/stop), Generate Info Signal/1(start/stop)
  Plant Input/1 -> Rate Transition2/1
  Plant Output/1 -> Rate Transition1/1
  Generate Ready Signal/1(Ready) -> Bus Creator1/1  "Ready"
  Subtract Nominal Values/2(PlantOutput) -> Bus Creator1/4  "PlantOutput"
  Subtract Nominal Values/1(PlantInput) -> Bus Creator1/3  "PlantInput"
  Rate Transition3/1 -> Bus Creator1/2, Generate Ready Signal/2(Perturbation)  "Perturbation"
  Bus Creator1/1 -> data/1
  Generate Info Signal/1(Info) -> Bus Creator1/5

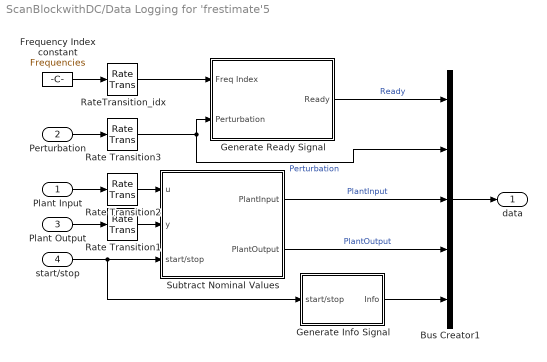
== system ScanBlockwithDC/Data Logging for 'frestimate'5 ==
  Plant Input : Inport
  Perturbation : Inport  Port=2
  Plant Output : Inport  Port=3
  start/stop : Inport  Port=4
  Bus Creator1 : BusCreator  Inputs=5
  Frequency Index constant : Constant  Value=Frequencies  OutDataTypeStr=double
  Generate Info Signal : Subsystem  Variant=on  VariantControlMode=label  LabelModeActiveChoice=VariantPRBS
  Generate Ready Signal : Subsystem  Variant=on  VariantControlMode=label  LabelModeActiveChoice=VariantPRBS
  Rate Transition1 : RateTransition  OutPortSampleTime=Ts
  Rate Transition2 : RateTransition  OutPortSampleTime=Ts
  Rate Transition3 : RateTransition  OutPortSampleTime=Ts
  RateTransition_idx : RateTransition  OutPortSampleTime=Ts
  Subtract Nominal Values : Subsystem
  data : Outport
  wires:
  Frequency Index constant/1 -> RateTransition_idx/1
  RateTransition_idx/1 -> Generate Ready Signal/1(Freq Index)
  Perturbation/1 -> Rate Transition3/1
  Rate Transition1/1 -> Subtract Nominal Values/2(y)
  Rate Transition2/1 -> Subtract Nominal Values/1(u)
  start/stop/1 -> Subtract Nominal Values/3(start/stop), Generate Info Signal/1(start/stop)
  Plant Input/1 -> Rate Transition2/1
  Plant Output/1 -> Rate Transition1/1
  Generate Ready Signal/1(Ready) -> Bus Creator1/1  "Ready"
  Subtract Nominal Values/2(PlantOutput) -> Bus Creator1/4  "PlantOutput"
  Subtract Nominal Values/1(PlantInput) -> Bus Creator1/3  "PlantInput"
  Rate Transition3/1 -> Bus Creator1/2, Generate Ready Signal/2(Perturbation)  "Perturbation"
  Bus Creator1/1 -> data/1
  Generate Info Signal/1(Info) -> Bus Creator1/5

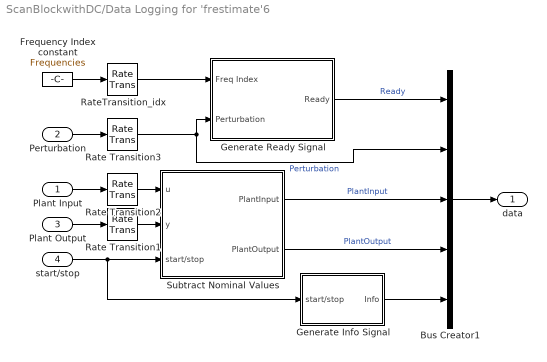
== system ScanBlockwithDC/Data Logging for 'frestimate'6 ==
  Plant Input : Inport
  Perturbation : Inport  Port=2
  Plant Output : Inport  Port=3
  start/stop : Inport  Port=4
  Bus Creator1 : BusCreator  Inputs=5
  Frequency Index constant : Constant  Value=Frequencies  OutDataTypeStr=double
  Generate Info Signal : Subsystem  Variant=on  VariantControlMode=label  LabelModeActiveChoice=VariantPRBS
  Generate Ready Signal : Subsystem  Variant=on  VariantControlMode=label  LabelModeActiveChoice=VariantPRBS
  Rate Transition1 : RateTransition  OutPortSampleTime=Ts
  Rate Transition2 : RateTransition  OutPortSampleTime=Ts
  Rate Transition3 : RateTransition  OutPortSampleTime=Ts
  RateTransition_idx : RateTransition  OutPortSampleTime=Ts
  Subtract Nominal Values : Subsystem
  data : Outport
  wires:
  Frequency Index constant/1 -> RateTransition_idx/1
  RateTransition_idx/1 -> Generate Ready Signal/1(Freq Index)
  Perturbation/1 -> Rate Transition3/1
  Rate Transition1/1 -> Subtract Nominal Values/2(y)
  Rate Transition2/1 -> Subtract Nominal Values/1(u)
  start/stop/1 -> Subtract Nominal Values/3(start/stop), Generate Info Signal/1(start/stop)
  Plant Input/1 -> Rate Transition2/1
  Plant Output/1 -> Rate Transition1/1
  Generate Ready Signal/1(Ready) -> Bus Creator1/1  "Ready"
  Subtract Nominal Values/2(PlantOutput) -> Bus Creator1/4  "PlantOutput"
  Subtract Nominal Values/1(PlantInput) -> Bus Creator1/3  "PlantInput"
  Rate Transition3/1 -> Bus Creator1/2, Generate Ready Signal/2(Perturbation)  "Perturbation"
  Bus Creator1/1 -> data/1
  Generate Info Signal/1(Info) -> Bus Creator1/5

== system ScanBlockwithDC/Sinusoidal Measurement (PLL, Three-Phase)1 ==
  note: Loop Filter (LF)
  note: Voltage-controlled oscillator (VCO)
  abc : Inport  PortDimensions=3  SampleTime=Ts
  Start/Stop : Inport  Port=2
  Angle : Subsystem
  Discrete : Subsystem  VariantControl=Discrete
      settings: LibrarySourceBlock=eeGeneralControl/Signal Sample and Hold/Discrete
  Low-Pass Filter (Discrete or Continuous) : eeGeneralControl/Low-Pass Filter (Discrete or Continuous)  K=1/2/pi  T=1e-3  B=inf  A=-inf  init_option=Specify as parameter  x0=F0  Ts=Ts
  Moving Average (Variable Frequency) : eeGeneralControl/Moving Average (Variable Frequency)  VariantControl=Variant1  LabelModeActiveChoice=Discrete  f0=F0  fmin=5  x0=0  BufferSize=8192  Ts=Ts
  PI : Subsystem
  Park Transform : eeTransforms/Park Transform  AxisAlignment=Q-axis  PowerInvariant=on
  Pythagorian Sum : Fcn  Expr=sqrt(u(1)^2+u(2)^2)
  Selector2 : Selector  InputPortWidth=3  IndexOptions=Index vector (dialog)  Indices=[2]  OutputSizes=1
  freq : Outport  VectorParamsAs1DForOutWhenUnconnected=off
  angle : Outport  Port=2  VectorParamsAs1DForOutWhenUnconnected=off
  mag : Outport  Port=3  VectorParamsAs1DForOutWhenUnconnected=off
  wires:
  Discrete/1(y) -> Angle/1(omega), Low-Pass Filter (Discrete or Continuous)/1
  PI/1(y) -> Discrete/1(u)
  Start/Stop/1 -> Discrete/2(S)
  Moving Average (Variable Frequency)/1 -> Selector2/1, Pythagorian Sum/1
  Selector2/1 -> PI/1(u)
  Low-Pass Filter (Discrete or Continuous)/1 -> freq/1, Moving Average (Variable Frequency)/1
  Angle/1(theta) -> angle/1, Park Transform/2
  Park Transform/1 -> Moving Average (Variable Frequency)/2
  Pythagorian Sum/1 -> mag/1
  abc/1 -> Park Transform/1

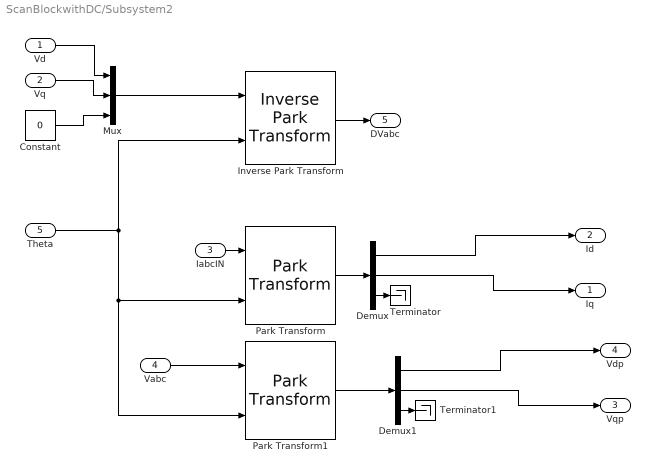
== system ScanBlockwithDC/Subsystem2 ==
  Vd : Inport
  Vq : Inport  Port=2
  IabcIN : Inport  Port=3
  Vabc : Inport  Port=4
  Theta : Inport  Port=5
  Constant : Constant  Value=0
  Demux : Demux  Outputs=3
  Demux1 : Demux  Outputs=3
  Inverse Park Transform : eeTransforms/Inverse Park Transform  AxisAlignment=Q-axis  PowerInvariant=on
  Mux : Mux  Inputs=3
  Park Transform : eeTransforms/Park Transform  AxisAlignment=Q-axis  PowerInvariant=on
  Park Transform1 : eeTransforms/Park Transform  AxisAlignment=Q-axis  PowerInvariant=on
  Terminator : Terminator
  Terminator1 : Terminator
  Iq : Outport
  Id : Outport  Port=2
  Vqp : Outport  Port=3
  Vdp : Outport  Port=4
  DVabc : Outport  Port=5
  wires:
  Constant/1 -> Mux/3
  Park Transform1/1 -> Demux1/1
  Demux1/2 -> Vqp/1
  Demux1/1 -> Vdp/1
  Demux1/3 -> Terminator1/1
  Vabc/1 -> Park Transform1/1
  Mux/1 -> Inverse Park Transform/1
  Demux/2 -> Iq/1
  Demux/1 -> Id/1
  Vd/1 -> Mux/1
  Park Transform/1 -> Demux/1
  Demux/3 -> Terminator/1
  Theta/1 -> Park Transform1/2, Park Transform/2, Inverse Park Transform/2
  Inverse Park Transform/1 -> DVabc/1
  IabcIN/1 -> Park Transform/1
  Vq/1 -> Mux/2

== system ScanBlockwithDC/Data Logging for 'frestimate'1/Generate Info Signal ==
  note: 1) Add Subsystem or Model blocks as valid variant choices.
      | 2) You cannot connect blocks at this level. At simulation, connectivity is automatically
      | determined, based on the active variant and port name matching.
  start/stop : Inport
  PRBS : Subsystem  VariantControl=VariantPRBS
  Sinestream : Subsystem  VariantControl=VariantSinestream
  Info : Outport

== system ScanBlockwithDC/Data Logging for 'frestimate'1/Generate Ready Signal ==
  note: 1) Add Subsystem or Model blocks as valid variant choices.
      | 2) You cannot connect blocks at this level. At simulation, connectivity is automatically
      | determined, based on the active variant and port name matching.
  Freq Index : Inport
  Perturbation : Inport  Port=2
  PRBS : Subsystem  VariantControl=VariantPRBS
  Sinestream : Subsystem  VariantControl=VariantSinestream
  Ready : Outport

== system ScanBlockwithDC/Data Logging for 'frestimate'1/Subtract Nominal Values ==
  u : Inport
  y : Inport  Port=2
  start/stop : Inport  Port=3
  Enabled Subsystem : Subsystem  TreatAsAtomicUnit=on
  PlantInput : Outport
  PlantOutput : Outport  Port=2
  wires:
  Enabled Subsystem/2(PlantOutput) -> PlantOutput/1
  Enabled Subsystem/1(PlantInput) -> PlantInput/1
  start/stop/1 -> Enabled Subsystem/Enable, Enabled Subsystem/3(start/stop)
  y/1 -> Enabled Subsystem/2(y)
  u/1 -> Enabled Subsystem/1(u)

== system ScanBlockwithDC/Data Logging for 'frestimate'2/Generate Info Signal ==
  note: 1) Add Subsystem or Model blocks as valid variant choices.
      | 2) You cannot connect blocks at this level. At simulation, connectivity is automatically
      | determined, based on the active variant and port name matching.
  start/stop : Inport
  PRBS : Subsystem  VariantControl=VariantPRBS
  Sinestream : Subsystem  VariantControl=VariantSinestream
  Info : Outport

== system ScanBlockwithDC/Data Logging for 'frestimate'2/Generate Ready Signal ==
  note: 1) Add Subsystem or Model blocks as valid variant choices.
      | 2) You cannot connect blocks at this level. At simulation, connectivity is automatically
      | determined, based on the active variant and port name matching.
  Freq Index : Inport
  Perturbation : Inport  Port=2
  PRBS : Subsystem  VariantControl=VariantPRBS
  Sinestream : Subsystem  VariantControl=VariantSinestream
  Ready : Outport

== system ScanBlockwithDC/Data Logging for 'frestimate'2/Subtract Nominal Values ==
  u : Inport
  y : Inport  Port=2
  start/stop : Inport  Port=3
  Enabled Subsystem : Subsystem  TreatAsAtomicUnit=on
  PlantInput : Outport
  PlantOutput : Outport  Port=2
  wires:
  Enabled Subsystem/2(PlantOutput) -> PlantOutput/1
  Enabled Subsystem/1(PlantInput) -> PlantInput/1
  start/stop/1 -> Enabled Subsystem/Enable, Enabled Subsystem/3(start/stop)
  y/1 -> Enabled Subsystem/2(y)
  u/1 -> Enabled Subsystem/1(u)

== system ScanBlockwithDC/Data Logging for 'frestimate'3/Generate Info Signal ==
  note: 1) Add Subsystem or Model blocks as valid variant choices.
      | 2) You cannot connect blocks at this level. At simulation, connectivity is automatically
      | determined, based on the active variant and port name matching.
  start/stop : Inport
  PRBS : Subsystem  VariantControl=VariantPRBS
  Sinestream : Subsystem  VariantControl=VariantSinestream
  Info : Outport

== system ScanBlockwithDC/Data Logging for 'frestimate'3/Generate Ready Signal ==
  note: 1) Add Subsystem or Model blocks as valid variant choices.
      | 2) You cannot connect blocks at this level. At simulation, connectivity is automatically
      | determined, based on the active variant and port name matching.
  Freq Index : Inport
  Perturbation : Inport  Port=2
  PRBS : Subsystem  VariantControl=VariantPRBS
  Sinestream : Subsystem  VariantControl=VariantSinestream
  Ready : Outport

== system ScanBlockwithDC/Data Logging for 'frestimate'3/Subtract Nominal Values ==
  u : Inport
  y : Inport  Port=2
  start/stop : Inport  Port=3
  Enabled Subsystem : Subsystem  TreatAsAtomicUnit=on
  PlantInput : Outport
  PlantOutput : Outport  Port=2
  wires:
  Enabled Subsystem/2(PlantOutput) -> PlantOutput/1
  Enabled Subsystem/1(PlantInput) -> PlantInput/1
  start/stop/1 -> Enabled Subsystem/Enable, Enabled Subsystem/3(start/stop)
  y/1 -> Enabled Subsystem/2(y)
  u/1 -> Enabled Subsystem/1(u)

== system ScanBlockwithDC/Data Logging for 'frestimate'4/Generate Info Signal ==
  note: 1) Add Subsystem or Model blocks as valid variant choices.
      | 2) You cannot connect blocks at this level. At simulation, connectivity is automatically
      | determined, based on the active variant and port name matching.
  start/stop : Inport
  PRBS : Subsystem  VariantControl=VariantPRBS
  Sinestream : Subsystem  VariantControl=VariantSinestream
  Info : Outport

== system ScanBlockwithDC/Data Logging for 'frestimate'4/Generate Ready Signal ==
  note: 1) Add Subsystem or Model blocks as valid variant choices.
      | 2) You cannot connect blocks at this level. At simulation, connectivity is automatically
      | determined, based on the active variant and port name matching.
  Freq Index : Inport
  Perturbation : Inport  Port=2
  PRBS : Subsystem  VariantControl=VariantPRBS
  Sinestream : Subsystem  VariantControl=VariantSinestream
  Ready : Outport

== system ScanBlockwithDC/Data Logging for 'frestimate'4/Subtract Nominal Values ==
  u : Inport
  y : Inport  Port=2
  start/stop : Inport  Port=3
  Enabled Subsystem : Subsystem  TreatAsAtomicUnit=on
  PlantInput : Outport
  PlantOutput : Outport  Port=2
  wires:
  Enabled Subsystem/2(PlantOutput) -> PlantOutput/1
  Enabled Subsystem/1(PlantInput) -> PlantInput/1
  start/stop/1 -> Enabled Subsystem/Enable, Enabled Subsystem/3(start/stop)
  y/1 -> Enabled Subsystem/2(y)
  u/1 -> Enabled Subsystem/1(u)

== system ScanBlockwithDC/Data Logging for 'frestimate'5/Generate Info Signal ==
  note: 1) Add Subsystem or Model blocks as valid variant choices.
      | 2) You cannot connect blocks at this level. At simulation, connectivity is automatically
      | determined, based on the active variant and port name matching.
  start/stop : Inport
  PRBS : Subsystem  VariantControl=VariantPRBS
  Sinestream : Subsystem  VariantControl=VariantSinestream
  Info : Outport

== system ScanBlockwithDC/Data Logging for 'frestimate'5/Generate Ready Signal ==
  note: 1) Add Subsystem or Model blocks as valid variant choices.
      | 2) You cannot connect blocks at this level. At simulation, connectivity is automatically
      | determined, based on the active variant and port name matching.
  Freq Index : Inport
  Perturbation : Inport  Port=2
  PRBS : Subsystem  VariantControl=VariantPRBS
  Sinestream : Subsystem  VariantControl=VariantSinestream
  Ready : Outport

== system ScanBlockwithDC/Data Logging for 'frestimate'5/Subtract Nominal Values ==
  u : Inport
  y : Inport  Port=2
  start/stop : Inport  Port=3
  Enabled Subsystem : Subsystem  TreatAsAtomicUnit=on
  PlantInput : Outport
  PlantOutput : Outport  Port=2
  wires:
  Enabled Subsystem/2(PlantOutput) -> PlantOutput/1
  Enabled Subsystem/1(PlantInput) -> PlantInput/1
  start/stop/1 -> Enabled Subsystem/Enable, Enabled Subsystem/3(start/stop)
  y/1 -> Enabled Subsystem/2(y)
  u/1 -> Enabled Subsystem/1(u)

== system ScanBlockwithDC/Data Logging for 'frestimate'6/Generate Info Signal ==
  note: 1) Add Subsystem or Model blocks as valid variant choices.
      | 2) You cannot connect blocks at this level. At simulation, connectivity is automatically
      | determined, based on the active variant and port name matching.
  start/stop : Inport
  PRBS : Subsystem  VariantControl=VariantPRBS
  Sinestream : Subsystem  VariantControl=VariantSinestream
  Info : Outport

== system ScanBlockwithDC/Data Logging for 'frestimate'6/Generate Ready Signal ==
  note: 1) Add Subsystem or Model blocks as valid variant choices.
      | 2) You cannot connect blocks at this level. At simulation, connectivity is automatically
      | determined, based on the active variant and port name matching.
  Freq Index : Inport
  Perturbation : Inport  Port=2
  PRBS : Subsystem  VariantControl=VariantPRBS
  Sinestream : Subsystem  VariantControl=VariantSinestream
  Ready : Outport

== system ScanBlockwithDC/Data Logging for 'frestimate'6/Subtract Nominal Values ==
  u : Inport
  y : Inport  Port=2
  start/stop : Inport  Port=3
  Enabled Subsystem : Subsystem  TreatAsAtomicUnit=on
  PlantInput : Outport
  PlantOutput : Outport  Port=2
  wires:
  Enabled Subsystem/2(PlantOutput) -> PlantOutput/1
  Enabled Subsystem/1(PlantInput) -> PlantInput/1
  start/stop/1 -> Enabled Subsystem/Enable, Enabled Subsystem/3(start/stop)
  y/1 -> Enabled Subsystem/2(y)
  u/1 -> Enabled Subsystem/1(u)
